simulink model "absorber_model"  (R2022a)
settings: Solver=VariableStepAuto  StartTime=0.0  StopTime=20  RelTol=1e-3
settings Model: Creator=Home  LastModifiedBy=Home

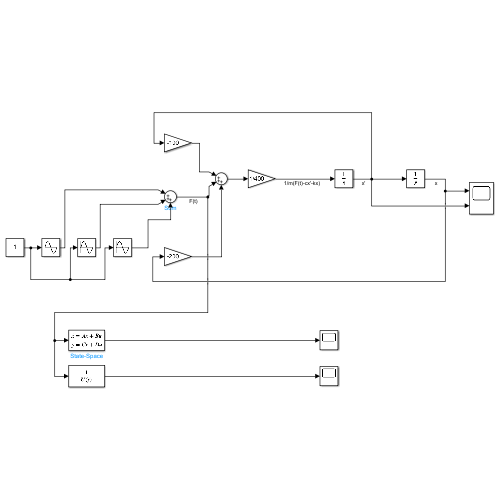
[thumbnail: Simulink's stored preview of the top-level diagram]
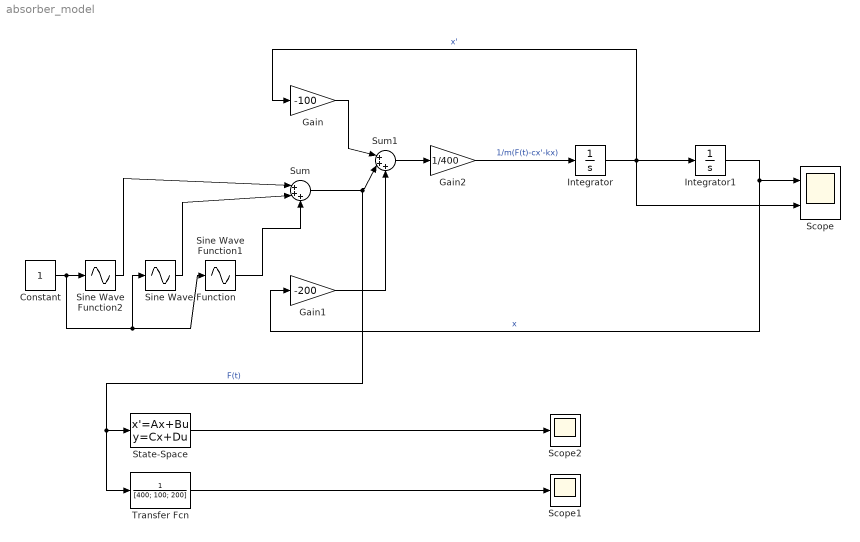
== system absorber_model ==
  Constant : Constant
  Gain : Gain  Gain=-100
  Gain1 : Gain  Gain=-200
  Gain2 : Gain  Gain=1/400
  Integrator : Integrator
  Integrator1 : Integrator
  Scope : Scope  NumInputPorts=2
  Scope1 : Scope
  Scope2 : Scope
  Sine Wave Function : Sin  TimeSource=Use external signal  Amplitude=10  Frequency=0.5  SampleTime=0
  Sine Wave Function1 : Sin  TimeSource=Use external signal  Amplitude=20  Frequency=1.5  SampleTime=0
  Sine Wave Function2 : Sin  TimeSource=Use external signal  Amplitude=50  Frequency=3  SampleTime=0
  State-Space : StateSpace  A=[0 1; -200/400 -100/400]  B=[0; 1/400]  C=[1 0]  D=0  InitialCondition=0  ParameterTunability=Unconstrained
  Sum : Sum  Inputs=|+++
  Sum1 : Sum  Inputs=|+++
  Transfer Fcn : TransferFcn  Denominator=[400; 100; 200]
  wires:
  Sine Wave Function2/1 -> Sum/1
  Sine Wave Function/1 -> Sum/2
  Sine Wave Function1/1 -> Sum/3
  Sum/1 -> Sum1/2, Transfer Fcn/1, State-Space/1  "F(t)"
  Gain/1 -> Sum1/1
  Gain1/1 -> Sum1/3
  Sum1/1 -> Gain2/1
  Integrator1/1 -> Gain1/1, Scope/1  "x"
  Integrator/1 -> Gain/1, Scope/2, Integrator1/1  "x'"
  Constant/1 -> Sine Wave Function1/1, Sine Wave Function/1, Sine Wave Function2/1
  State-Space/1 -> Scope2/1
  Transfer Fcn/1 -> Scope1/1
  Gain2/1 -> Integrator/1  "1/m(F(t)-cx'-kx)"
